simulink model "P6"  (R2024b)
settings: Solver=VariableStepAuto  StartTime=0.0  StopTime=.01  RelTol=1e-3
InitFcn:
  | L=.002;
  | R=10;
  | C=.00001;

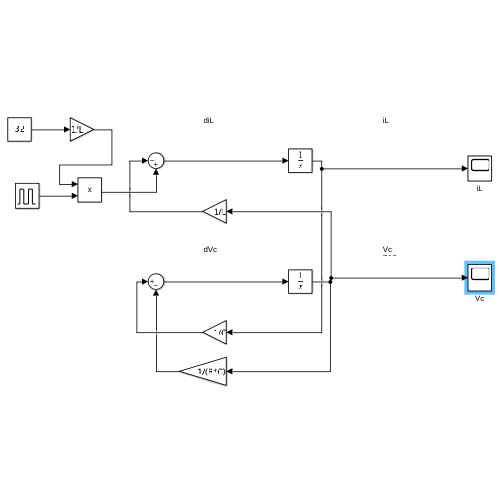
[thumbnail: Simulink's stored preview of the top-level diagram]
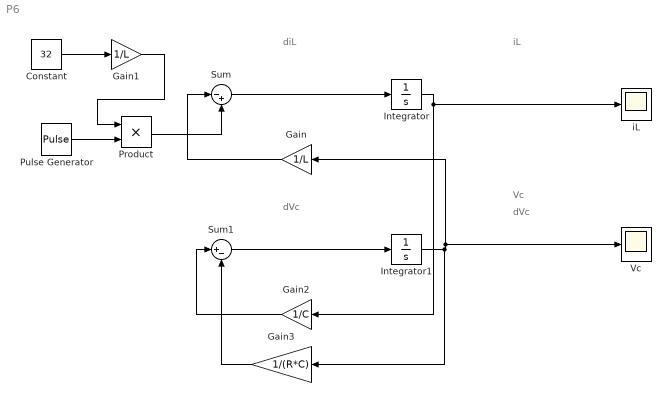
== system P6 ==
  note: diL
  note: iL
  note: dVc
  note: dVc
  note: Vc
  Constant : Constant  Value=32
  Gain : Gain  Gain=1/L
  Gain1 : Gain  Gain=1/L
  Gain2 : Gain  Gain=1/C
  Gain3 : Gain  Gain=1/(R*C)
  Integrator : Integrator
  Integrator1 : Integrator
  Product : Product
  Pulse Generator : DiscretePulseGenerator  PulseType=Time based  Amplitude=.955  Period=.00001  PulseWidth=40
  Sum : Sum  Inputs=|-+
  Sum1 : Sum  Inputs=|+-
  Vc : Scope
  iL : Scope
  wires:
  Sum/1 -> Integrator/1
  Sum1/1 -> Integrator1/1
  Gain/1 -> Sum/1
  Integrator1/1 -> Gain3/1, Gain/1, Vc/1
  Constant/1 -> Gain1/1
  Gain1/1 -> Product/1
  Product/1 -> Sum/2
  Integrator/1 -> iL/1, Gain2/1
  Gain2/1 -> Sum1/1
  Gain3/1 -> Sum1/2
  Pulse Generator/1 -> Product/2
